simulink model "Extension1"  (R2023a)
settings: Solver=VariableStepAuto  StartTime=0.0  StopTime=1  RelTol=1e-3
InitFcn:
  | Lab2Rob
values from neighbouring files (symbols this model uses):
  A = [0, 0, 1, 0 ... (first row only)    [InitialCons.m]    (also in Lab3Rob.m; LinearizeA.m = [0,0,1,0;0,0,0,1;0,-(l*m*g*(J+m*r^2+m^2+l*M*m))/(I*J+J*L^2*M; xaMatrix.m)
  B = [ ... (first row only)    [InitialCons.m]    (also in Lab3Rob.m; LinearizeB.m)
  K = lqr(A,B,Q,R)    [Lab3Rob.m]
  qdq = [0;2;0;0]    [InitialCons.m]
settings Model: Creator=willi  LastModifiedBy=willi

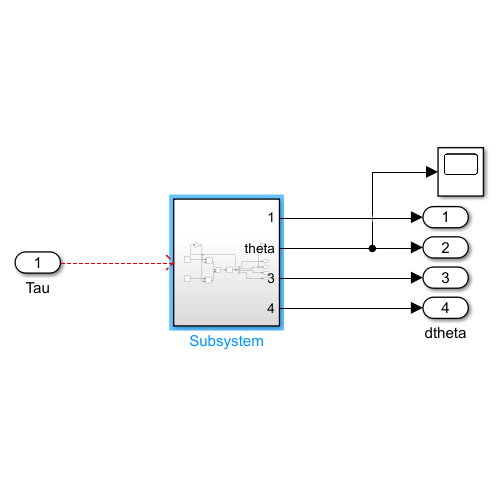
[thumbnail: Simulink's stored preview of the top-level diagram]
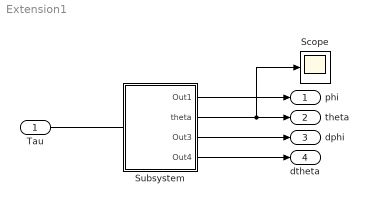
== system Extension1 ==
  Tau : Inport
  Scope : Scope
  Subsystem : Subsystem
  phi : Outport
  theta : Outport  Port=2
  dphi : Outport  Port=3
  dtheta : Outport  Port=4
  wires:
  Tau/1 -> ?
  Subsystem/1(Out1) -> phi/1
  Subsystem/3(Out3) -> dphi/1
  Subsystem/4(Out4) -> dtheta/1
  Subsystem/2(theta) -> Scope/1, theta/1

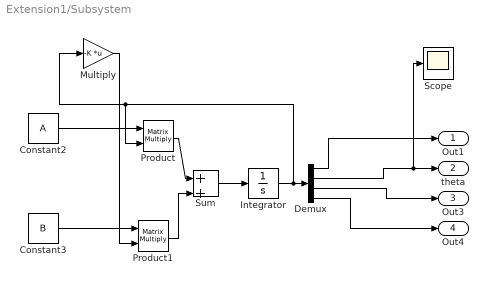
== system Extension1/Subsystem ==
  Constant2 : Constant  Value=A  VectorParams1D=off
  Constant3 : Constant  Value=B
  Demux : Demux
  Integrator : Integrator  InitialCondition=qdq
  Multiply : Gain  Gain=-K  Multiplication=Matrix(K*u)
  Product : Product  Multiplication=Matrix(*)
  Product1 : Product  Multiplication=Matrix(*)
  Scope : Scope
  Sum : Sum  Inputs=|++
  Out1 : Outport
  theta : Outport  Port=2
  Out3 : Outport  Port=3
  Out4 : Outport  Port=4
  wires:
  Demux/3 -> Out3/1
  Constant3/1 -> Product1/1
  Product1/1 -> Sum/2
  Sum/1 -> Integrator/1
  Product/1 -> Sum/1
  Demux/4 -> Out4/1
  Integrator/1 -> Multiply/1, Product/2, Demux/1
  Constant2/1 -> Product/1
  Demux/2 -> Scope/1, theta/1
  Demux/1 -> Out1/1
  Multiply/1 -> Product1/2
